simulink model "PV_JEINC"  (Simulink 10.2)
settings: Solver=FixedStepAuto  StartTime=0.0  StopTime=0.3  FixedStep=1e-6  RelTol=1e-3
libraries: powerlib x17, re_lib x4, powerlib_meascontrol x1
settings Model: Creator=11383  LastModifiedBy=Administrator  SimulationMode=accelerator
settings DataIOCC: SaveFormat=Dataset  SignalLoggingSaveFormat=Dataset
settings OptimizationCC: LifeSpan=auto
settings DebuggingCC: UnderspecifiedInitializationDetection=Simplified  MergeDetectMultiDrivingBlocksExec=error  FcnCallInpInsideContextMsg=error  SFUnexpectedBacktrackingDiag=error  SFNoUnconditionalDefaultTransitionDiag=error  SFExecutionAtInitializationDiag=warning
settings HardwareCC: ProdBitPerPointer=64  ProdBitPerSizeT=64  ProdBitPerPtrDiffT=64  ProdLargestAtomicFloat=Float  ProdIntDivRoundTo=Zero  ProdEndianess=LittleEndian  ProdWordSize=64  ProdHWDeviceType=Intel->x86-64 (Windows64)
settings ModelReferenceCC: PropagateSignalLabelsOutOfModel=on
settings GRTTargetCC: TargetLangStandard=C99 (ISO)  CombineOutputUpdateFcns=on  GRTInterface=off
settings ConfigComp: CovMetricSettings=dwe  CovSaveCumulativeToWorkspaceVar=off  CovSaveSingleToWorkspaceVar=off  CovExternalEMLEnable=on
settings SimscapeCC: SimscapeNormalizeSystem=off

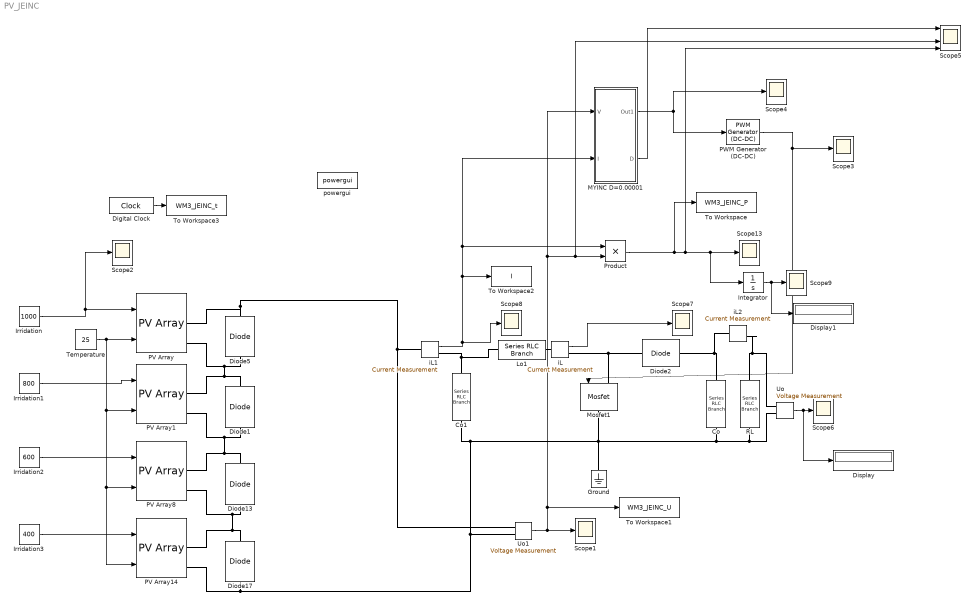
== system PV_JEINC ==
  Co : powerlib/Elements/Series RLC Branch  LConnTagsString=__new0  RConnTagsString=__new0  BranchType=C  Resistance=1e-4  Inductance=50e-3  SetiL0=off  InitialCurrent=0  Capacitance=9e-5  Setx0=off  InitialVoltage=0  Measurements=None
  Co1 : powerlib/Elements/Series RLC Branch  LConnTagsString=__new0  RConnTagsString=__new0  BranchType=C  Resistance=1e-4  Inductance=50e-3  SetiL0=off  InitialCurrent=0  Capacitance=200e-5  Setx0=off  InitialVoltage=0  Measurements=None
  Digital Clock : DigitalClock  SampleTime=-1
  Diode{1,5,13,17} (4 alike) : powerlib/Power Electronics/Diode  Ron=0.001  Lon=0  Vf=0.8  IC=0  UseSnubber=off  Rs=inf  Cs=250e-9  Measurements=off
  Diode2 : powerlib/Power Electronics/Diode  Ron=0.001  Lon=0  Vf=0.001  IC=0  UseSnubber=off  Rs=inf  Cs=inf  Measurements=off
  Display : Display
  Display1 : Display
  Ground : powerlib/Elements/Ground  LConnTagsString=a
  Integrator : Integrator
  Irridation : Constant  Value=1000  SampleTime=0.001
  Irridation1 : Constant  Value=800  SampleTime=0.001
  Irridation2 : Constant  Value=600  SampleTime=0.001
  Irridation3 : Constant  Value=400  SampleTime=0.001
  Lo1 : powerlib/Elements/Series RLC Branch  LConnTagsString=__new0  RConnTagsString=__new0  BranchType=L  Resistance=0.1  Inductance=2e-3  SetiL0=off  InitialCurrent=0  Capacitance=1e-12  Setx0=off  InitialVoltage=0  Measurements=None
  MYINC D=0.00001 : Subsystem
  Mosfet1 : powerlib/Power Electronics/Mosfet  Ron=0.001  Lon=0  Rd=0.0001  Vfd=0  IC=0  Rs=1e8  Cs=inf  Measurements=off
  PV Array{,1,8,14} (4 alike) : re_lib/Solar/PV Array  Npar=1  Nser=1  PlotType=array @ 1000 W/m2 & specified temperatures  S_vec="[ 1000  500  100 ]"  Temp_C_vec="[ 45 25  ]"  ModuleName=User-defined  PlotWhenSelected=off  Pm=120.75  Ncell=16  Voc=22  Isc=7.5  Vm=17.5  Im=6.9  beta_Voc_pc=-0.36099  alpha_Isc_pc=0.102  beta_Voc=-0.079418  alpha_Isc=0.00765  IL=7.6829  I0=2.1898e-10  nI=2.2089  Rsh=50.0358  Rs=0.26399  RobustModel=off  RobustCellTemperature=313.3991  BAL=off  Tc=1e-6  Tfilter=5e-5
  PWM Generator (DC-DC) : powerlib_meascontrol/Pulse & Signal Generators/PWM Generator (DC-DC)  Fsw=10000  Ts=5e-6
  Product : Product
  RL : powerlib/Elements/Series RLC Branch  LConnTagsString=__new0  RConnTagsString=__new0  BranchType=R  Resistance=33  Inductance=50e-3  SetiL0=off  InitialCurrent=0  Capacitance=1e-12  Setx0=off  InitialVoltage=0  Measurements=None
  Scope{1..4,6..9,13} (9 alike) : Scope
  Scope5 : Scope  NumInputPorts=4
  Temperature : Constant  Value=25  SampleTime=0.001
  To Workspace : ToWorkspace  VariableName=WM3_JEINC_P  SampleTime=-1
  To Workspace1 : ToWorkspace  VariableName=WM3_JEINC_U  SampleTime=-1
  To Workspace2 : ToWorkspace  VariableName=I  SampleTime=-1
  To Workspace3 : ToWorkspace  VariableName=WM3_JEINC_t  SampleTime=-1
  Uo : powerlib/Measurements/Voltage Measurement  PhasorSimulation=off  OutputType=Complex  PSBequivalent=0
  Uo1 : powerlib/Measurements/Voltage Measurement  PhasorSimulation=off  OutputType=Complex  PSBequivalent=0
  iL : powerlib/Measurements/Current Measurement  PhasorSimulation=off  OutputType=Complex  PSBequivalent=0
  iL1 : powerlib/Measurements/Current Measurement  PhasorSimulation=off  OutputType=Complex  PSBequivalent=0
  iL2 : powerlib/Measurements/Current Measurement  PhasorSimulation=off  OutputType=Complex  PSBequivalent=0
  powergui : powerlib/powergui  SimulationMode=Discrete  SampleTime=1e-6  frequency=60  Iterations=50  frequencyindice=0  Pbase=100e6  ErrMax=1e-4  UnitsV=kV  UnitsW=MW  buscounter=0  FunctionMessages=off  echomessages=off  EnableUseOfTLC=off  CurrentSourceSwitches=off  DisableSnubberDevices=off  DisableRonSwitches=off  DisableVfSwitches=off  DisplayEquations=off  AutomaticDiscreteSolvers=off  SolverType=Tustin  Interpol=off  ExternalGateDelay=off  methode=off  Ts=0  x0status=blocks  SPID=off  SwTol=0  HookPort=off  NonlinearTolerance=0  nMaxIteration=15  ContinueOnMaxIteration=off  RestoreLinks=warning  ResistiveCurrentMeasurement=off  Frange=[0:2:500]  Ylog=off  Xlog=on  ShowGrid=off  save=off  variable=ZData  structure=0  ZoomFFT=on  StartTime=0.0  cycles=1  DisplayStyle=1  fundamental=60  FreqAxis=off  MaxFrequency=1000  frequencyindicesteady=1  RmsSteady=1  display=off
  wires:
  Uo/1 -> Display/1, Scope6/1
  PWM Generator (DC-DC)/1 -> Mosfet1/1, Scope3/1
  MYINC D=0.00001/1(Out1) -> Scope4/1, PWM Generator (DC-DC)/1
  Product/1 -> To Workspace/1, Integrator/1, Scope13/1, Scope5/4
  Uo1/1 -> To Workspace1/1, MYINC D=0.00001/1("V "), Scope5/3, Product/2, Scope1/1
  iL/1 -> Scope7/1
  iL1/1 -> Scope8/1, To Workspace2/1, MYINC D=0.00001/2(I), Product/1
  Temperature/1 -> PV Array14/2, PV Array8/2, PV Array1/2, PV Array/2
  Irridation/1 -> PV Array/1, Scope2/1
  MYINC D=0.00001/2(D) -> Scope5/1
  Irridation1/1 -> PV Array1/1
  Irridation2/1 -> PV Array8/1
  Irridation3/1 -> PV Array14/1
  Integrator/1 -> Display1/1, Scope9/1
  Digital Clock/1 -> To Workspace3/1
  connections:
  Uo/LConn1 -- iL2/RConn1 -- RL/RConn1
  Mosfet1/LConn1 -- Diode2/LConn1 -- iL/RConn1
  iL1/RConn1 -- Co1/LConn1 -- Lo1/LConn1
  Uo1/LConn1 -- PV Array/RConn1 -- Diode5/RConn1 -- iL1/LConn1
  Uo1/LConn2 -- PV Array14/RConn2 -- Diode17/LConn1 -- Mosfet1/RConn1 -- Ground/LConn1 -- Co/RConn1 -- RL/LConn1 -- Uo/LConn2 -- Co1/RConn1
  iL/LConn1 -- Lo1/RConn1
  Co/LConn1 -- iL2/LConn1 -- Diode2/RConn1
  PV Array8/RConn2 -- Diode13/LConn1 -- Diode17/RConn1 -- PV Array14/RConn1
  PV Array1/RConn1 -- Diode5/LConn1 -- PV Array/RConn2 -- Diode1/RConn1
  PV Array1/RConn2 -- Diode1/LConn1 -- Diode13/RConn1 -- PV Array8/RConn1

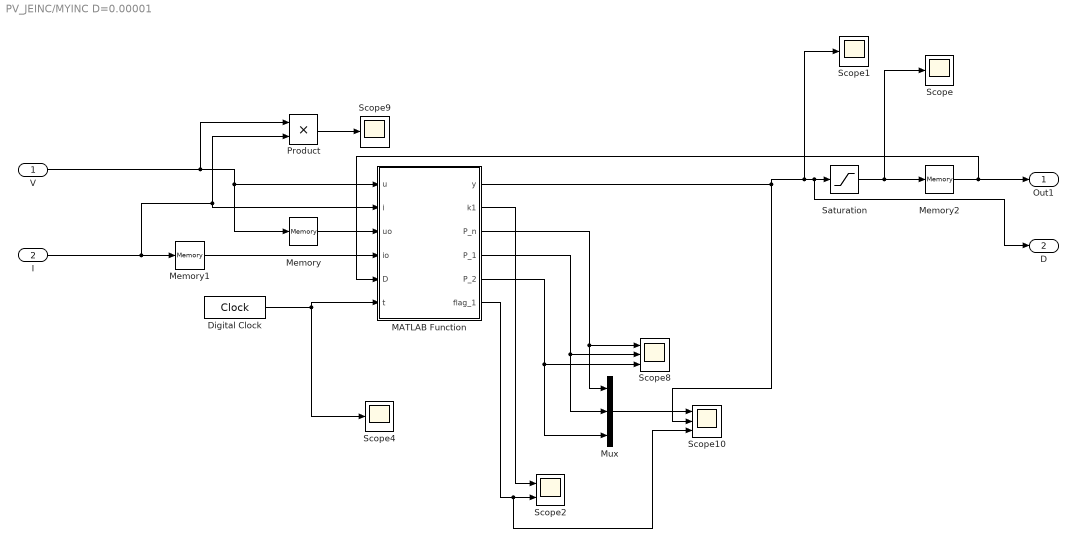
== system PV_JEINC/MYINC D=0.00001 ==
  "V " : Inport
  I : Inport  Port=2
  Digital Clock : DigitalClock  SampleTime=-1
  MATLAB Function : MATLAB Function  TreatAsAtomicUnit=on
  Memory : Memory
  Memory1 : Memory
  Memory2 : Memory
  Mux : Mux  Inputs=3
  Product : Product
  Saturation : Saturate  UpperLimit=0.9  LowerLimit=0.1
  Scope{,1,4,9} (4 alike) : Scope
  Scope10 : Scope  NumInputPorts=3
  Scope2 : Scope  NumInputPorts=2
  Scope8 : Scope  NumInputPorts=3
  Out1 : Outport  VectorParamsAs1DForOutWhenUnconnected=off
  D : Outport  Port=2  VectorParamsAs1DForOutWhenUnconnected=off
  wires:
  "V "/1 -> Product/1, Memory/1, MATLAB Function/1(u)
  Memory/1 -> MATLAB Function/3(uo)
  I/1 -> Memory1/1, Product/2, MATLAB Function/2(i)
  Memory1/1 -> MATLAB Function/4(io)
  Memory2/1 -> MATLAB Function/5(D), Out1/1
  MATLAB Function/1(y) -> Scope1/1, D/1, Saturation/1, Scope10/2
  Saturation/1 -> Scope/1, Memory2/1
  Digital Clock/1 -> Scope4/1, MATLAB Function/6(t)
  MATLAB Function/2(k1) -> Scope2/1
  MATLAB Function/3(P_n) -> Mux/1, Scope8/1
  MATLAB Function/4(P_1) -> Mux/2, Scope8/2
  MATLAB Function/5(P_2) -> Mux/3, Scope8/3
  Product/1 -> Scope9/1
  Mux/1 -> Scope10/1
  MATLAB Function/6(flag_1) -> Scope10/3, Scope2/2

== matlab function MYINC D=0.00001/MATLAB Function ==
  data: u input double; y output double; i input double; uo input double; io input double; D input double; t input double; k1 output double; P_n output double; P_1 output double; P_2 output double; flag_1 output double
function [y,k1,P_n,P_1,P_2,flag_1]= JEINC(u,i,uo,io,D,t)
%% Parameters Initialization
m=0;
P=u*i;
du=u-uo;
di=i-io;
dp=(u*i)-(uo*io);
A=1;
d=0.01*A;
h=0;
%% 稳态判断
persistent T; %稳态前两步采样时间控制量
if isempty(T)
    T=0.001;
end
persistent P1; %存储前两步对比用的功率值
if isempty(P1)
    P1=0;
end
persistent P2; %采样前一步对比用的功率值
if isempty(P2)
    P2=0;
end
persistent D1; %存储前两步对比用的功率值
if isempty(D1)
    D1=0;
end
persistent D2; %存储前两步对比用的功率值
if isempty(D2)
    D2=0;
end
persistent Pn; %采样前一步对比用的功率值
if isempty(Pn)
    Pn=0;
end
persistent flag; %进入稳态次数
if isempty(flag)
    flag=1;
end
persistent Pmax; %更新最大功率值
if isempty(Pmax)
    Pmax=0;
end
persistent Xmax; %更新最大功率值对应占空比
if isempty(Xmax)
    Xmax=0;
end
persistent Ts; %更新最大功率值对应占空比
if isempty(Ts)
    Ts=0;
end
%% 位置更新参数
x=[0.2 0.4 0.6 0.8];
persistent k;   %稳态次数标识符
if isempty(k) 
    k=1;
end
% if abs(t-T)<0.001
%     P1=P2;
%     P2=u*i;
%     T=T+0.001;
% end 
% T_scope=T;
% deltaP=abs(P1-P2);
%% 采样
sam_p = rem(t,T);  %sample_point 对t信号除以T取余，余数为0，返回值0
if(sam_p==0)
P2=P1;
P1=Pn;
Pn=P;
% else
%     sin_s = sin_n;
%     sin_s1 = sin_p1;
%     sin_s2 = sin_p2;
end
% sin_n = sin_s;

   
D2=D1;
D1=D;


%% Algorithm
error1=Pn-P1;
error2=P1-P2;
if  error1*error2<0 && flag<5 %判断是否进入稳定状态
    m=0;

    if abs(D2-D1)>(2*d)
        k=k+1;
        if (k<6)
            flag = k;
        end
    end
else %不满足重启条件，则进入INC
    if du==0
        if di==0
            m=D;
        else
            if di>0
                m=D-d;
            else
                m=D+d;
            end
        end
    else
        if di/du== -(i/u)
            m=D;
        else
            if di/du> -(i/u)
                m=D-d;
            else
                m=D+d;
            end
        end
    end
end
%% 最优位置更新
if P>Pmax               %如果某一点的P值大于最优值的话
    Xmax=D;             %把更高的P值对应的电压值赋给最优值
    Pmax=P;             %把更高的P值赋给最优值
end
%% 输出占空比
y = m;
k1=k;
P_n=Pn;
P_1=P1;
P_2=P2;
flag_1=flag;
end
